simulink model "circular_data"  (R2024b)
settings: Solver=ode4  StartTime=0.0  StopTime=simulation_time  FixedStep=sample_time  RelTol=1e-3
values from neighbouring files (symbols this model uses):
  init_dq = initial(i).init_dq    [LyaOrder8.m]
  init_q = initial(i).init_q    [LyaOrder8.m]
settings Model: Creator=zhes  LastModifiedBy=zhes

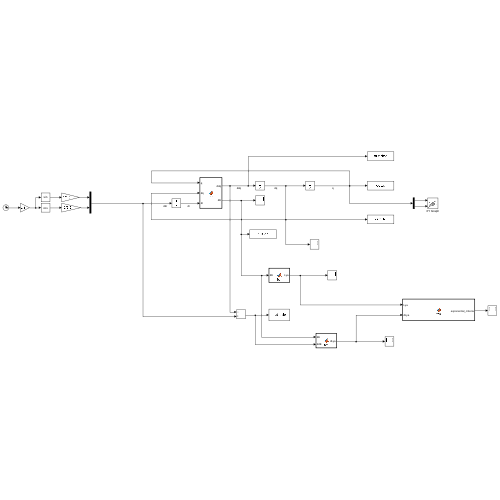
[thumbnail: Simulink's stored preview of the top-level diagram]
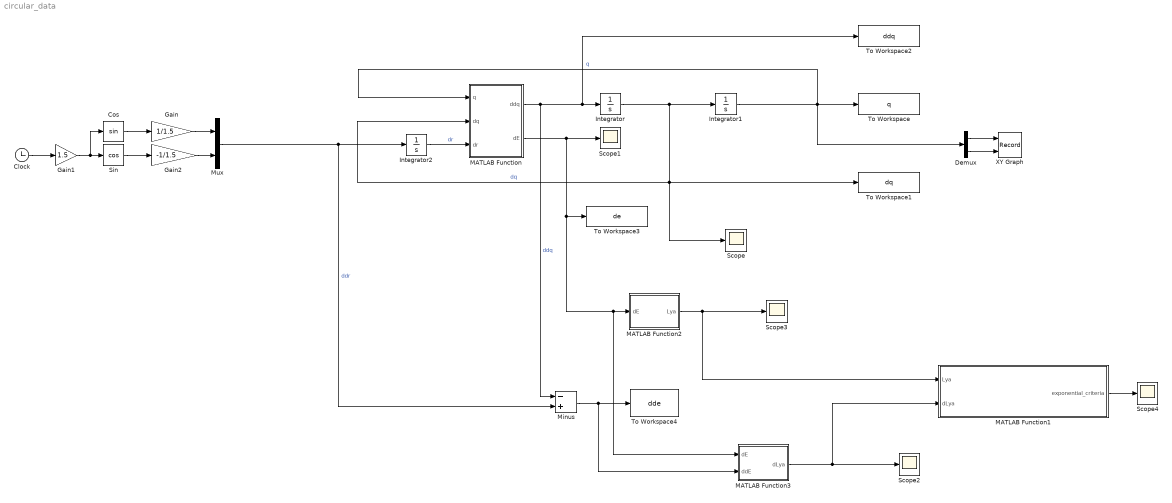
== system circular_data ==
  Clock : Clock
  Cos : Trigonometry
  Demux : Demux  Outputs=2
  Gain : Gain  Gain=1/1.5
  Gain1 : Gain  Gain=1.5
  Gain2 : Gain  Gain=-1/1.5
  Integrator : Integrator  InitialCondition=init_dq
  Integrator1 : Integrator  InitialCondition=init_q
  Integrator2 : Integrator  InitialCondition=[ 1 ; 1 ]
  MATLAB Function : MATLAB Function  TreatAsAtomicUnit=on
  MATLAB Function1 : MATLAB Function  TreatAsAtomicUnit=on
  MATLAB Function2 : MATLAB Function  TreatAsAtomicUnit=on
  MATLAB Function3 : MATLAB Function  TreatAsAtomicUnit=on
  Minus : Sum  Inputs=-+
  Mux : Mux  Inputs=2
  Scope{,1..4} (5 alike) : Scope
  Sin : Trigonometry  Operator=cos
  To Workspace : ToWorkspace  VariableName=q  SaveFormat=Structure With Time  SampleTime=-1
  To Workspace1 : ToWorkspace  VariableName=dq  SaveFormat=Structure With Time  SampleTime=-1
  To Workspace2 : ToWorkspace  VariableName=ddq  SaveFormat=Structure With Time  SampleTime=-1
  To Workspace3 : ToWorkspace  VariableName=de  SaveFormat=Structure With Time  SampleTime=-1
  To Workspace4 : ToWorkspace  VariableName=dde  SaveFormat=Structure With Time  SampleTime=-1
  XY Graph : Record  FileSettingsInternal="{\"entries\":[{\"content\":{\"excelSettings\":{\"content\":{},\"type\":\"Streamout.ExcelSettings\"}},\"type\":\"Streamout.FileSettingStorage\",\"uuid\":\"\"}],\"packageUris\":[\"http:\\/\\/schema.mathworks.com\\/mf0\\/streamout_blocks\\/R2020a\"],\"version\":\"1.0\"}"  Layout=[1 1]  SignalsInternal="{\"entries\":[{\"content\":{\"signals\":[{\"content\":{\"blockPath\":[],\"dimensions\":[1,1],\"domain\":\"\",\"lineColor\":\"#a2142f\",\"plots\":[ 1 ],\"port\":1,\"sid\":[\"\"],\"signalID\":1,\"signalName\":\"Demux:1\"},\"type\":\"RecordBlkView.Signal\",\"uuid\":\"\"},{\"content\":{\"blockPath\":[],\"dimensions\":[1,1],\"domain\":\"\",\"lineColor\":\"#139fff\",\"plots\":[ 1 ],\"port\":2,\"sid\":[\"\"],\"signalID\":2,\"signalName\":\"Demux:2\"},\"type\":\"RecordBlkView.Signal\",\"uuid\":\"\"}]},\"type\":\"RecordBlkView.InputSignals\",\"uuid\":\"\"}],\"packageUris\":[\"http:\\/\\/schema.mathworks.com\\/mf0\\/streamout_blocks\\/R2020a\"],\"version\":\"1.0\"}"  VisualizationBindings="{\"xyplotplugin\":{\"info\":[{\"series\":[{\"bindingParametersList\":[{\"parameter\":\"X-Axis\",\"signalID\":1,\"signalName\":\"Demux:1\"},{\"parameter\":\"Y-Axis\",\"signalID\":2,\"signalName\":\"Demux:2\"}],\"seriesID\":0}],\"subplotID\":1}]}}"  CompatibilityTag=XY
  wires:
  Integrator/1 -> MATLAB Function/2(dq), To Workspace1/1, Scope/1, Integrator1/1  "dq"
  Integrator1/1 -> MATLAB Function/1(q), Demux/1, To Workspace/1  "q"
  MATLAB Function/1(ddq) -> Minus/1, To Workspace2/1, Integrator/1  "ddq"
  Integrator2/1 -> MATLAB Function/3(dr)  "dr"
  MATLAB Function/2(dE) -> MATLAB Function3/1(dE), MATLAB Function2/1(dE), To Workspace3/1, Scope1/1
  Mux/1 -> Integrator2/1, Minus/2  "ddr"
  Minus/1 -> MATLAB Function3/2(ddE), To Workspace4/1
  Sin/1 -> Gain2/1
  Gain1/1 -> Cos/1, Sin/1
  Clock/1 -> Gain1/1
  Cos/1 -> Gain/1
  Gain/1 -> Mux/1
  Gain2/1 -> Mux/2
  MATLAB Function2/1(Lya) -> MATLAB Function1/1(Lya), Scope3/1
  MATLAB Function1/1(exponential_criteria) -> Scope4/1
  MATLAB Function3/1(dLya) -> MATLAB Function1/2(dLya), Scope2/1
  Demux/2 -> XY Graph/2
  Demux/1 -> XY Graph/1

== matlab function circular_data/MATLAB Function1 ==
  data: Lya input; exponential_criteria output; dLya input
function exponential_criteria = fcn(Lya, dLya)

lambda = 0.0010;

exponential_criteria = dLya - lambda * Lya;

== matlab function circular_data/MATLAB Function ==
  data: q input; ddq output; dq input; dr input; dE output
function [ddq, dE]= fcn(q, dq, dr)

q1 = q(1);
q2 = q(2);
dq1 = dq(1);
dq2 = dq(2);

dr1 = dr(1);
dr2 = dr(2);

kD = diag([10,10]);

de1 = dr1 - dq1;
de2 = dr2 - dq2;

dE = [de1; de2];

ddq = kD * dE;

== matlab function circular_data/MATLAB Function2 ==
  data: dE input; Lya output
function Lya = fcn(dE)

de1 = dE(1);
de2 = dE(2);

a = [    0.0000
   -0.0000
    0.0001
   -0.0004
   -0.0009
   -0.0023
    0.0020
   -0.0073
    0.0076
   -0.0366
   -0.0289
    0.0053
    0.0604
    0.1913
    0.5596
   -0.4624
   -0.4183
    0.7022
    0.3438
    1.0884
    0.1973
   -1.0071
    0.7831
    0.7829
    0.4554
    0.4893
    0.5329
   -0.2303
    0.3277
   -0.6510
    0.3997
   -0.9226
   -0.4537
   -0.9117
   -0.7446
    0.6456
    0.3978
   -0.3645
    0.9026
   -0.9304
   -0.1228
   -0.2378
    0.0010 ];

Lya = ...
    a(1) * de1^2 + a(2) * de2^2 + a(3) * de1 * de2 + ...
    a(4) * de1^3 + a(5) * de2^3 + a(6) * de1^2 * de2 + a(7) * de1 * de2^2 + ...
    a(8) * de1^4 + a(9) * de2^4 + a(10) * de1^3 * de2 + a(11) * de1 * de2^3 + a(12) * de1^2 * de2^2 + ...
    a(13) * de1^5 + a(14) * de2^5 + a(15) * de1^4 * de2 + a(16) * de1 * de2^4 + a(17) * de1^3 * de2^2 + a(18) * de1^2 * de2^3 + ...
    a(19) * de1^6 + a(20) * de2^6 + a(21) * de1^5 * de2 + a(22) * de1 * de2^5 + a(23) * de1^4 * de2^2 + a(24) * de1^2 * de2^4 + a(25) * de1^3 * de2^3 + ...
    a(26) * de1^7 + a(27) * de2^7 + a(28) * de1^6 * de2 + a(29) * de1 * de2^6 + a(30) * de1^5 * de2^2 + a(31) * de1^2 * de2^5 + a(32) * de1^4 * de2^3 + a(33) * de1^3 * de2^4 + ...
    a(34) * de1^8 + a(35) * de2^8 + a(36) * de1^7 * de2 + a(37) * de1 * de2^7 + a(38) * de1^6 * de2^2 + a(39) * de1^2 * de2^6 + a(40) * de1^5 * de2^3 + a(41) * de1^3 * de2^5 + a(42) * de1^4 * de2^4;

== matlab function circular_data/MATLAB Function3 ==
  data: dE input; dLya output; ddE input
function dLya = fcn(dE, ddE)

de1 = dE(1);
de2 = dE(2);

dde1 = ddE(1);
dde2 = ddE(2);


a = [    0.0000
   -0.0000
    0.0001
   -0.0004
   -0.0009
   -0.0023
    0.0020
   -0.0073
    0.0076
   -0.0366
   -0.0289
    0.0053
    0.0604
    0.1913
    0.5596
   -0.4624
   -0.4183
    0.7022
    0.3438
    1.0884
    0.1973
   -1.0071
    0.7831
    0.7829
    0.4554
    0.4893
    0.5329
   -0.2303
    0.3277
   -0.6510
    0.3997
   -0.9226
   -0.4537
   -0.9117
   -0.7446
    0.6456
    0.3978
   -0.3645
    0.9026
   -0.9304
   -0.1228
   -0.2378
    0.0010 ];




gradient_Lya = [8*a(34)*de1^7 + 7*a(36)*de1^6*de2 + 7*a(26)*de1^6 + 6*a(38)*de1^5*de2^2 + 6*a(28)*de1^5*de2 + 6*a(19)*de1^5 + 5*a(40)*de1^4*de2^3 + 5*a(30)*de1^4*de2^2 + 5*a(21)*de1^4*de2 + 5*a(13)*de1^4 + 4*a(42)*de1^3*de2^4 + 4*a(32)*de1^3*de2^3 + 4*a(23)*de1^3*de2^2 + 4*a(15)*de1^3*de2 + 4*a(8)*de1^3 + 3*a(41)*de1^2*de2^5 + 3*a(33)*de1^2*de2^4 + 3*a(25)*de1^2*de2^3 + 3*a(17)*de1^2*de2^2 + 3*a(10)*de1^2*de2 + 3*a(4)*de1^2 + 2*a(39)*de1*de2^6 + 2*a(31)*de1*de2^5 + 2*a(24)*de1*de2^4 + 2*a(18)*de1*de2^3 + 2*a(12)*de1*de2^2 + 2*a(6)*de1*de2 + 2*a(1)*de1 + a(37)*de2^7 + a(29)*de2^6 + a(22)*de2^5 + a(16)*de2^4 + a(11)*de2^3 + a(7)*de2^2 + a(3)*de2, a(36)*de1^7 + 2*a(38)*de1^6*de2 + a(28)*de1^6 + 3*a(40)*de1^5*de2^2 + 2*a(30)*de1^5*de2 + a(21)*de1^5 + 4*a(42)*de1^4*de2^3 + 3*a(32)*de1^4*de2^2 + 2*a(23)*de1^4*de2 + a(15)*de1^4 + 5*a(41)*de1^3*de2^4 + 4*a(33)*de1^3*de2^3 + 3*a(25)*de1^3*de2^2 + 2*a(17)*de1^3*de2 + a(10)*de1^3 + 6*a(39)*de1^2*de2^5 + 5*a(31)*de1^2*de2^4 + 4*a(24)*de1^2*de2^3 + 3*a(18)*de1^2*de2^2 + 2*a(12)*de1^2*de2 + a(6)*de1^2 + 7*a(37)*de1*de2^6 + 6*a(29)*de1*de2^5 + 5*a(22)*de1*de2^4 + 4*a(16)*de1*de2^3 + 3*a(11)*de1*de2^2 + 2*a(7)*de1*de2 + a(3)*de1 + 8*a(35)*de2^7 + 7*a(27)*de2^6 + 6*a(20)*de2^5 + 5*a(14)*de2^4 + 4*a(9)*de2^3 + 3*a(5)*de2^2 + 2*a(2)*de2];


dLya = gradient_Lya * [dde1; dde2];
